simulink model "MODELLING_CONTROL_QUADCOPTER"  (R2023b)
settings: Solver=VariableStepAuto  StartTime=0.0  StopTime=120  FixedStep=0.018  RelTol=1e-3
undefined symbols (not defined in the file): D, drag_gain, gravity, Kf, Km, mass, mass_load, waypoints
libraries: slpidlib x8, matrix_library x4, shared6dof x1, sim3dlib x1, uavsim3dlib x1
(part 2 of 2)

== matlab function MODELLING_CONTROL_QUADCOPTER/MATLAB Function ==
  settings: updateMethod=DISCRETE
  data: Waypoints input; X_target output; CurrentPos input; Y_target output; Z_target output; done output; Tolerance input
function [X_target, Y_target, Z_target, done] = waypointTracker(Waypoints, CurrentPos, Tolerance)
    % Inputs:
    % Waypoints: Nx3 matris (X, Y, Z)
    % CurrentPos: 1x3 vektör (X, Y, Z)
    % Tolerance: Waypoint'e ulaşım toleransı
    
    persistent currentIndex;
    if isempty(currentIndex)
        currentIndex = 1;
    end
    
    % Aktif waypoint'i al
    X_target = Waypoints(currentIndex, 1);
    Y_target = Waypoints(currentIndex, 2);
    Z_target = Waypoints(currentIndex, 3);
   
    
    % Hata hesapla
    error = sqrt((CurrentPos(1) - X_target)^2 + ...
                 (CurrentPos(2) - Y_target)^2 + ...
                 (CurrentPos(3) - Z_target)^2);
    
    % Waypoint'e ulaşıldıysa bir sonrakine geç
    if error < Tolerance
        currentIndex = currentIndex + 1;
    end
    
    % Tüm waypoints bitti mi?
    if currentIndex > size(Waypoints, 1)
        done = true; % Simülasyonu bitir
        currentIndex = size(Waypoints, 1); % Son waypoint'te kal
    else
        done = false;
    end
end

== matlab function MODELLING_CONTROL_QUADCOPTER/disturbances/MATLAB Function2 ==
  data: velocity input; Frain output
function Frain = rainDrag(velocity)
    Cd_rain = 0.05;  % Yağmur altındaki sürükleme katsayısı
    Frain = -Cd_rain * velocity;  % hıza ters yönlü lineer drag
end

== matlab function MODELLING_CONTROL_QUADCOPTER/disturbances/MATLAB Function3 ==
  data: t input; Fw output; Mw output
function [Fw, Mw] = windDisturbance(t)
    % Sinüs dalgası ile değişen rüzgar kuvvetleri
    Fx = 0.2 * sin(0.3*t);  % X yönü rüzgarı
    Fy = 0.3 * sin(0.5*t + pi/4);  % Y yönü rüzgarı
    Fz = 0;  % Z yönünde rüzgar sabit ya da ihmal edilebilir

    Mx = 0.01 * sin(0.4*t);
    My = 0.01 * cos(0.6*t);
    Mz = 0.005 * sin(0.2*t);

    Fw = [Fx; Fy; Fz];
    Mw = [Mx; My; Mz];
end

== matlab function MODELLING_CONTROL_QUADCOPTER/Sensors/MATLAB Function ==
  data: t input; x input; x_s output; y input; z input; roll input; pitch input; yaw input; y_s output; z_s output; roll_s output; pitch_s output; yaw_s output
function [x_s, y_s, z_s, roll_s, pitch_s, yaw_s] = sensorSmokeEffect(t, x, y, z, roll, pitch, yaw)
% Simulates time-varying sensor disturbances due to smoke effects

% --- Position bias (constant)
bias_xyz = [0.05, -0.03, 0.04]; % meters

% --- Position noise (time-varying with sine modulation)
noise_xyz = 0.02 * sin(0.5 * t + [0, 1, 2]);  % small noise in x, y, z

x_s = x + bias_xyz(1) + noise_xyz(1);
y_s = y + bias_xyz(2) + noise_xyz(2);
z_s = z + bias_xyz(3) + noise_xyz(3);

% --- RPY bias (constant)
bias_rpy = deg2rad([1.0, -0.5, 0.7]);  % radians

% --- RPY noise (time-varying)
noise_rpy = deg2rad(0.3 * cos(0.4 * t + [0, 2, 4]));

roll_s  = roll  + bias_rpy(1) + noise_rpy(1);
pitch_s = pitch + bias_rpy(2) + noise_rpy(2);
yaw_s   = yaw   + bias_rpy(3) + noise_rpy(3);
end
